simulink model "theme4"  (R2025b)
settings: Solver=ode45  StartTime=0.0  StopTime=4  MaxStep=1e-5  MinStep=1e-6  RelTol=1e-3
settings Model: Creator=ktrog  LastModifiedBy=ktrog
settings SolverCC: InitialStep=1e-5

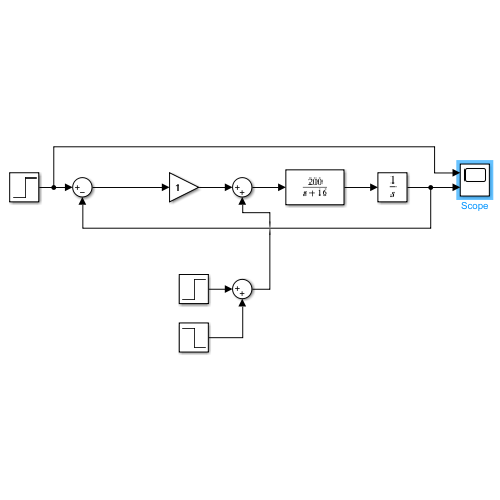
[thumbnail: Simulink's stored preview of the top-level diagram]
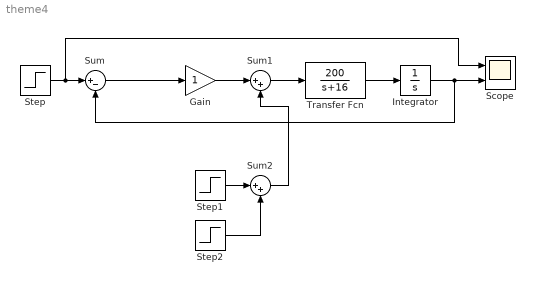
== system theme4 ==
  Gain : Gain
  Integrator : Integrator
  Scope : Scope  NumInputPorts=2
      settings: ActiveDisplayYMinimum=-0.47376226805213939  ActiveDisplayYMaximum=1.8556292367983529
  Step : Step  Time=0  SampleTime=0
  Step1 : Step  Time=2  SampleTime=0
  Step2 : Step  Time=2.1  After=-1  SampleTime=0
  Sum : Sum  Inputs=|+-
  Sum1 : Sum  Inputs=|++
  Sum2 : Sum  Inputs=|++
  Transfer Fcn : TransferFcn  Numerator=[200]  Denominator=[1 16]
  wires:
  Step/1 -> Scope/1, Sum/1
  Sum/1 -> Gain/1
  Gain/1 -> Sum1/1
  Sum1/1 -> Transfer Fcn/1
  Transfer Fcn/1 -> Integrator/1
  Integrator/1 -> Scope/2, Sum/2
  Step1/1 -> Sum2/1
  Step2/1 -> Sum2/2
  Sum2/1 -> Sum1/2
